simulink model "easy_sliding_mode_2"  (R2019b)
settings: Solver=VariableStepAuto  StartTime=0.0  StopTime=10.0  RelTol=1e-3
settings Model: Creator=Alien  LastModifiedBy=Alien

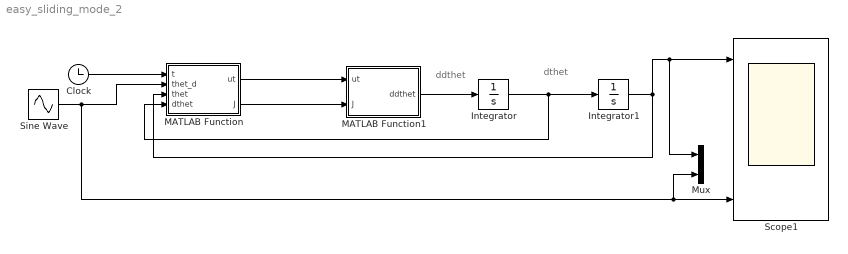
== system easy_sliding_mode_2 ==
  note: dthet
  note: ddthet
  Clock : Clock
  Integrator : Integrator  InitialCondition=5
  Integrator1 : Integrator  InitialCondition=2.5
  MATLAB Function : MATLAB Function  TreatAsAtomicUnit=on
  MATLAB Function1 : MATLAB Function  TreatAsAtomicUnit=on
  Mux : Mux  Inputs=2
  Scope1 : Scope  NumInputPorts=5
  Sine Wave : Sin  Amplitude=5  SampleTime=0
  wires:
  Integrator/1 -> MATLAB Function/4(dthet), Integrator1/1
  MATLAB Function1/1(ddthet) -> Integrator/1
  MATLAB Function/1(ut) -> MATLAB Function1/1(ut)
  MATLAB Function/2(J) -> MATLAB Function1/2(J)
  Integrator1/1 -> Mux/1, Scope1/1, MATLAB Function/3(thet)
  Clock/1 -> MATLAB Function/1(t)
  Sine Wave/1 -> Mux/2, Scope1/5, MATLAB Function/2(thet_d)

== matlab function easy_sliding_mode_2/MATLAB Function1 ==
  data: ut input; ddthet output; J input
function ddthet = fcn(ut,J)
ddthet = (1/J)*ut;
end

== matlab function easy_sliding_mode_2/MATLAB Function ==
  data: t input; ut output; thet_d input; thet input; dthet input; J output
function [ut,J] = fcn(t,thet_d,thet,dthet)
j = 10;
nta = 0.5;
c = 0.5;
dthet_d = cos(t);
ddthet_d = -sin(t);
e = thet-thet_d;
de = dthet - dthet_d;
s = c*e + de;
ut = j*(c*de+ddthet_d-nta*sign(s));
J = j;
end
